simulink model "model_reg"  (R2024a)
settings: Solver=FixedStepAuto  StartTime=0.0  StopTime=10  FixedStep=0.0001  MinStep=1e-8  RelTol=1e-8  AbsTol=1e-8
model workspace (MAT data in the model file):
  A = [11  -2  13; 6  -1  6; -6  -1  -8]
  B = [2; 0; 0]
  K = [-4 2.4167 -3]
values from neighbouring files (symbols this model uses):
  K1_1 = Y*inv(P)    [reg1.m]
  K1_2 = Y*inv(P)    [reg2.m]
  K1_3 = Y*inv(P)    [reg3.m]
  K2_1 = Y*inv(P)    [reg_minimize1.m]
  K2_2 = Y*inv(P)    [reg_minimize2.m]
  K2_3 = Y*inv(P)    [reg_minimize3.m]
settings Model: Creator=ventus  LastModifiedBy=ventus

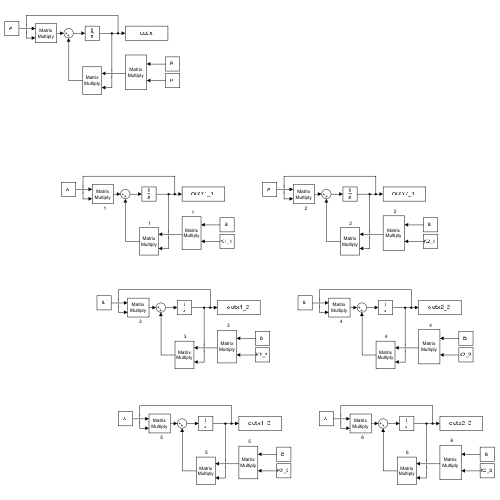
[thumbnail: Simulink's stored preview of the top-level diagram]
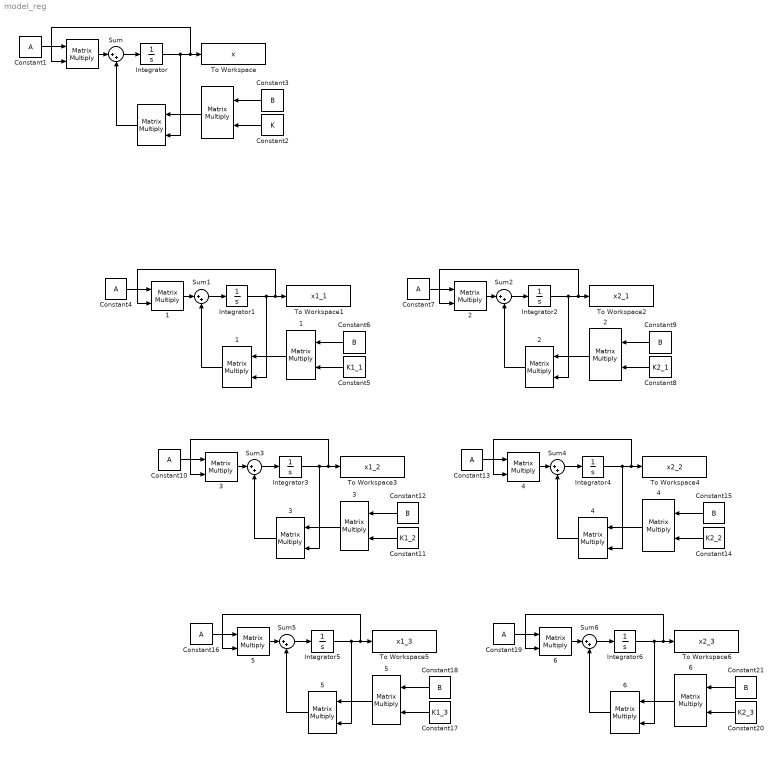
== system model_reg ==
   {,1..6} (7 alike) : Product  Multiplication=Matrix(*)
    {,1..6} (7 alike) : Product  Multiplication=Matrix(*)
     {,1..6} (7 alike) : Product  Multiplication=Matrix(*)
  Constant{1,4,7,10,13,16,19} (7 alike) : Constant  Value=A  VectorParams1D=off
  Constant11 : Constant  Value=K1_2  VectorParams1D=off
  Constant{3,6,9,12,15,18,21} (7 alike) : Constant  Value=B  VectorParams1D=off
  Constant14 : Constant  Value=K2_2  VectorParams1D=off
  Constant17 : Constant  Value=K1_3  VectorParams1D=off
  Constant2 : Constant  Value=K  VectorParams1D=off
  Constant20 : Constant  Value=K2_3  VectorParams1D=off
  Constant5 : Constant  Value=K1_1  VectorParams1D=off
  Constant8 : Constant  Value=K2_1  VectorParams1D=off
  Integrator{,1..6} (7 alike) : Integrator  InitialCondition=[1; 1; 1]
  Sum{,1..6} (7 alike) : Sum  Inputs=|++
  To Workspace : ToWorkspace  VariableName=x  SaveFormat=Timeseries  SampleTime=-1
  To Workspace1 : ToWorkspace  VariableName=x1_1  SaveFormat=Timeseries  SampleTime=-1
  To Workspace2 : ToWorkspace  VariableName=x2_1  SaveFormat=Timeseries  SampleTime=-1
  To Workspace3 : ToWorkspace  VariableName=x1_2  SaveFormat=Timeseries  SampleTime=-1
  To Workspace4 : ToWorkspace  VariableName=x2_2  SaveFormat=Timeseries  SampleTime=-1
  To Workspace5 : ToWorkspace  VariableName=x1_3  SaveFormat=Timeseries  SampleTime=-1
  To Workspace6 : ToWorkspace  VariableName=x2_3  SaveFormat=Timeseries  SampleTime=-1
  wires:
  Integrator/1 -> To Workspace/1, "   "/2, " "/2
  Constant2/1 -> "  "/2
  "  "/1 -> " "/1
  " "/1 -> Sum/2
  Sum/1 -> Integrator/1
  Constant3/1 -> "  "/1
  Constant1/1 -> "   "/1
  "   "/1 -> Sum/1
  " 1"/1 -> Sum1/2
  Constant6/1 -> "  1"/1
  "  1"/1 -> " 1"/1
  "   1"/1 -> Sum1/1
  Sum1/1 -> Integrator1/1
  Constant4/1 -> "   1"/1
  Constant5/1 -> "  1"/2
  Integrator1/1 -> To Workspace1/1, "   1"/2, " 1"/2
  " 2"/1 -> Sum2/2
  Constant9/1 -> "  2"/1
  "  2"/1 -> " 2"/1
  "   2"/1 -> Sum2/1
  Sum2/1 -> Integrator2/1
  Constant7/1 -> "   2"/1
  Constant8/1 -> "  2"/2
  Integrator2/1 -> To Workspace2/1, "   2"/2, " 2"/2
  "  4"/1 -> " 4"/1
  Integrator3/1 -> To Workspace3/1, "   3"/2, " 3"/2
  Constant14/1 -> "  4"/2
  Integrator4/1 -> To Workspace4/1, "   4"/2, " 4"/2
  "   4"/1 -> Sum4/1
  "  3"/1 -> " 3"/1
  Constant13/1 -> "   4"/1
  " 3"/1 -> Sum3/2
  Constant15/1 -> "  4"/1
  "   3"/1 -> Sum3/1
  Sum4/1 -> Integrator4/1
  " 4"/1 -> Sum4/2
  Constant12/1 -> "  3"/1
  Constant11/1 -> "  3"/2
  Sum3/1 -> Integrator3/1
  Constant10/1 -> "   3"/1
  "  6"/1 -> " 6"/1
  Integrator5/1 -> To Workspace5/1, "   5"/2, " 5"/2
  Constant20/1 -> "  6"/2
  Integrator6/1 -> To Workspace6/1, "   6"/2, " 6"/2
  "   6"/1 -> Sum6/1
  "  5"/1 -> " 5"/1
  Constant19/1 -> "   6"/1
  " 5"/1 -> Sum5/2
  Constant21/1 -> "  6"/1
  "   5"/1 -> Sum5/1
  Sum6/1 -> Integrator6/1
  " 6"/1 -> Sum6/2
  Constant18/1 -> "  5"/1
  Constant17/1 -> "  5"/2
  Sum5/1 -> Integrator5/1
  Constant16/1 -> "   5"/1
